simulink model "DC_Motor"  (R2016a)
settings: Solver=VariableStepAuto  StartTime=0.0  StopTime=100.0  RelTol=1e-3
values from neighbouring files (symbols this model uses):
  b = 3.5077E-6    [data.sldd]
  J = 3.2284E-6    [data.sldd]
  ke = 0.0274    [data.sldd]
  kt = 0.0274    [data.sldd]
  L = 2.75E-6    [data.sldd]
  R = 4.0    [data.sldd]
settings Model: DataDictionary=data.sldd  Creator=Admin  LastModifiedBy=Admin
settings DataIOCC: SaveOutput=off  SaveTime=off

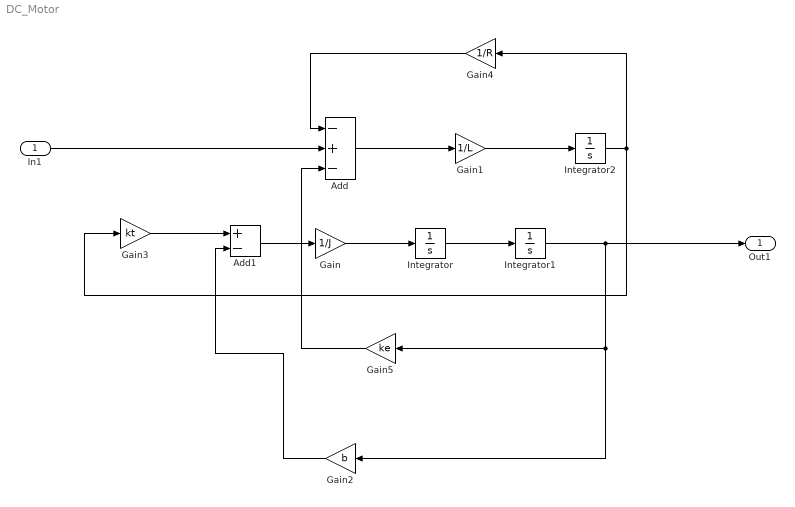
== system DC_Motor ==
  In1 : Inport  OutDataTypeStr=double  PortDimensions=1  SampleTime=0
  Add : Sum  Inputs=-+-
  Add1 : Sum  Inputs=+-
  Gain : Gain  Gain=1/J
  Gain1 : Gain  Gain=1/L
  Gain2 : Gain  Gain=b
  Gain3 : Gain  Gain=kt
  Gain4 : Gain  Gain=1/R
  Gain5 : Gain  Gain=ke
  Integrator : Integrator
  Integrator1 : Integrator
  Integrator2 : Integrator
  Out1 : Outport  OutDataTypeStr=double  PortDimensions=1  SampleTime=0
  wires:
  Integrator1/1 -> Gain2/1, Gain5/1, Out1/1
  Gain/1 -> Integrator/1
  Gain3/1 -> Add1/1
  Gain1/1 -> Integrator2/1
  Add1/1 -> Gain/1
  In1/1 -> Add/2
  Integrator2/1 -> Gain4/1, Gain3/1
  Gain2/1 -> Add1/2
  Gain4/1 -> Add/1
  Integrator/1 -> Integrator1/1
  Add/1 -> Gain1/1
  Gain5/1 -> Add/3
